simulink model "MRAC_IAI"  (R2020a)
settings: Solver=FixedStepAuto  StartTime=0.0  StopTime=20  FixedStep=0.01  RelTol=1e-3
InitFcn:
  | variableLoad
values from neighbouring files (symbols this model uses):
  a = 1    [variableLoad.m]
  a_ampl = 10    [variableLoad.m]
  a_m = -1    [variableLoad.m]
  a_varFreq = 1/10    (= 0.1)    [variableLoad.m]
undefined symbols (not defined in the file or in its folder): b
libraries: cstblocks x1
settings Model: Creator=alfystar  LastModifiedBy=emanu

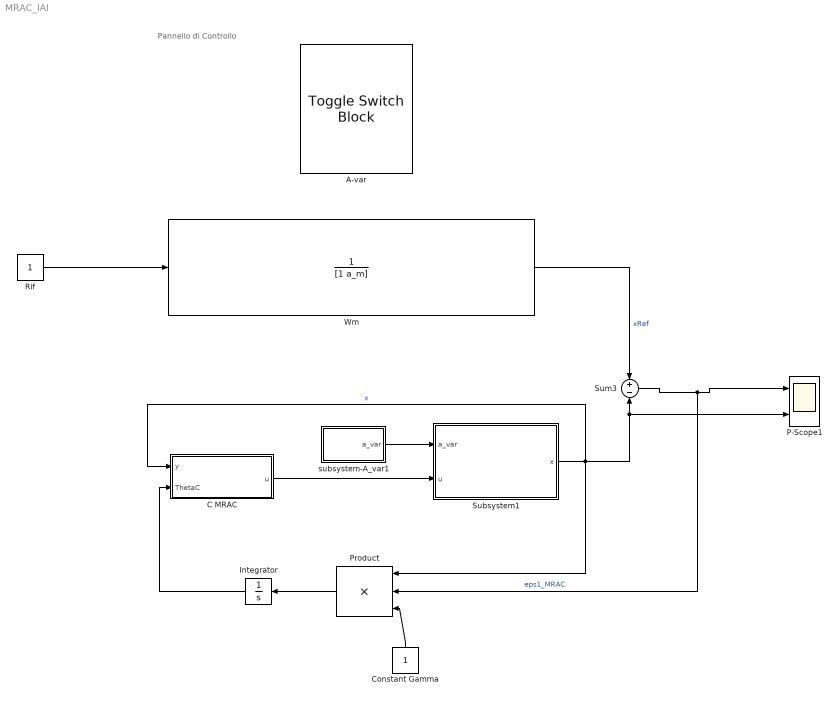
== system MRAC_IAI ==
  note: Pannello di Controllo
  "A-var " : ToggleSwitchBlock  LabelPosition=Hide
      settings: Values={{'TimeVariant-Off', 'TimeVariant-On'}, [0 1]}
  C MRAC : MATLAB Function  TreatAsAtomicUnit=on
  Constant Gamma : Constant
  Integrator : Integrator
  P-Scope1 : Scope  NumInputPorts=2
  Product : Product  Inputs=3
  Rif : Constant
  Subsystem1 : Subsystem
  Sum3 : Sum  Inputs=+|-
  Wm : TransferFcn  Denominator=[1 a_m]
  subsystem-A_var1 : Subsystem
  wires:
  subsystem-A_var1/1(a_var) -> Subsystem1/1(a_var)
  C MRAC/1(u) -> Subsystem1/2(u)
  Wm/1 -> Sum3/1  "xRef"
  Subsystem1/1(x) -> Product/1, C MRAC/1(y), P-Scope1/2, Sum3/2  "x"
  Sum3/1 -> Product/2, P-Scope1/1  "eps1_MRAC"
  Constant Gamma/1 -> Product/3
  Product/1 -> Integrator/1
  Integrator/1 -> C MRAC/2(ThetaC)
  Rif/1 -> Wm/1

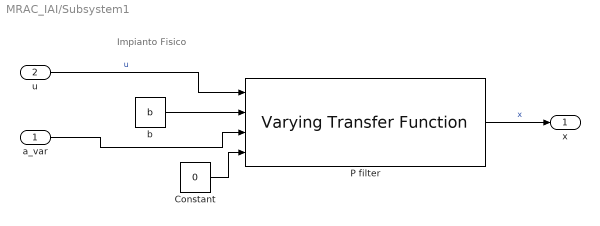
== system MRAC_IAI/Subsystem1 ==
  note: Impianto Fisico
  a_var : Inport
  u : Inport  Port=2
  Constant : Constant  Value=0
  P filter : cstblocks/Linear Parameter Varying/Varying Transfer Function  N=1
  b : Constant  Value=b
  x : Outport
  wires:
  P filter/1 -> x/1  "x"
  u/1 -> P filter/1  "u"
  a_var/1 -> P filter/3
  Constant/1 -> P filter/4
  b/1 -> P filter/2

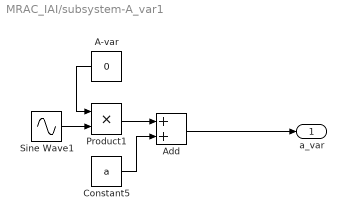
== system MRAC_IAI/subsystem-A_var1 ==
  A-var : Constant  Value=0
  Add : Sum
  Constant5 : Constant  Value=a
  Product1 : Product
  Sine Wave1 : Sin  Amplitude=a_ampl  Frequency=a_varFreq  SampleTime=0
  a_var : Outport
  wires:
  Constant5/1 -> Add/2
  Add/1 -> a_var/1
  Sine Wave1/1 -> Product1/2
  A-var/1 -> Product1/1
  Product1/1 -> Add/1

== matlab function MRAC_IAI/C MRAC ==
  data: y input; u output; ThetaC input
function u = C(y,ThetaC)

u=-y*ThetaC;

end
